simulink model "DRI_furnace"  (R2023b)
settings: Solver=ode15s  StartTime=0.0  StopTime=3600*24
values from neighbouring files (symbols this model uses):
  a_b = 6*(1-eps_bed)/(r_p*2)    (= 200)    [DRI_furnace_loader.m]
  A_furnace = pi*r_furnace^2    (= 23.7582944428)    [DRI_furnace_loader.m]
  A_furnace_pel = A_furnace*(1-eps_bed)    (= 11.8791472214)    [DRI_furnace_loader.m]
  A_wall = (2*pi*r_furnace*dz)    [DRI_furnace_loader.m]
  c_CH4init = interp1([1:1:length(c_CH4init)],c_CH4init, linspace(1,length(c_CH4init),n_furnace))    [DRI_furnace_loader.m]    (also in inital_conditions.m = out.CH4_conc.data(end,:); initcond.mat = [1.85705986545 1.89555733619 1.89749367615 1.89250716351 1.8; initcond_H2.mat = [-5.10200321778e-23 -5.14631233267e-23 -5.19105613109e-23 -5; initcond_NG.mat = [1.53547326032 1.50495486962 1.48970115024 1.4755028102 1.46)
  c_Cinit = interp1([1:1:length(c_Cinit)],c_Cinit, linspace(1,length(c_Cinit),n_furnace))    [DRI_furnace_loader.m]    (also in inital_conditions.m = out.C_conc.data(end,:); initcond.mat = [3.21457388191e-26 -1.33944556404e-26 -9.41053781484e-33 -9.; initcond_H2.mat = [-3.07981965757e-283 -7.05821276017e-284 -1.12151880238e-284; initcond_NG.mat = [40.5707549093 38.5039319297 36.8451113121 35.2570306703 33.)
  c_CO2init = interp1([1:1:length(c_CO2init)],c_CO2init, linspace(1,length(c_CO2init),n_furnace))    [DRI_furnace_loader.m]    (also in inital_conditions.m = out.CO2_conc.data(end,:); initcond.mat = [0.424855142623 0.487573768012 0.610878568601 0.778581871411; initcond_H2.mat = [8.08256932825e-22 8.11925418298e-22 8.15917924386e-22 8.201; initcond_NG.mat = [0.33936960913 0.362161667495 0.389241162314 0.417886502664 )
  c_COinit = interp1([1:1:length(c_COinit)],c_COinit, linspace(1,length(c_COinit),n_furnace))    [DRI_furnace_loader.m]    (also in inital_conditions.m = out.CO_conc.data(end,:); initcond.mat = [5.62429774676 5.68698007947 5.56998267729 5.3860363993 5.16; initcond_H2.mat = [-3.5707332813e-22 -3.59888147715e-22 -3.62743836785e-22 -3.; initcond_NG.mat = [7.01547259829 7.0384402498 7.00998897858 6.97797046171 6.94)
  c_Fe2O3init = interp1([1:1:length(c_Fe2O3init)],c_Fe2O3init, linspace(1,length(c_Fe2O3init),n_furnace))    [DRI_furnace_loader.m]    (also in inital_conditions.m = out.Fe2O3_conc.data(end,:); initcond.mat = [845.154140842 845.181508816 845.220501809 845.323312901 845; initcond_H2.mat = [-0.0380770099519 -0.0370367139242 -0.0360185883395 -0.03502; initcond_NG.mat = [-0.0405281021674 -0.0396025120519 -0.0386898228266 -0.03778)
  c_Fe3O4init = interp1([1:1:length(c_Fe3O4init)],c_Fe3O4init, linspace(1,length(c_Fe3O4init),n_furnace))    [DRI_furnace_loader.m]    (also in inital_conditions.m = out.Fe3O4_conc.data(end,:); initcond.mat = [826.123395955 826.094631755 826.211564736 834.377927258 899; initcond_H2.mat = [0.0321426182211 0.0314818734285 0.030826675132 0.0301767421; initcond_NG.mat = [0.0360465051239 0.0353534026747 0.0346647730928 0.033980211)
  c_Feinit = interp1([1:1:length(c_Feinit)],c_Feinit, linspace(1,length(c_Feinit),n_furnace))    [DRI_furnace_loader.m]    (also in inital_conditions.m = out.Fe_conc.data(end,:); initcond.mat = [836.997845525 830.524010614 758.675200979 644.11637995 545.; initcond_H2.mat = [2198.89990701 2151.53921086 2100.32127816 2045.76128409 198; initcond_NG.mat = [2217.04023267 2190.22219582 2162.02573698 2132.25158626 210)
  c_FeOinit = interp1([1:1:length(c_FeOinit)],c_FeOinit, linspace(1,length(c_FeOinit),n_furnace))    [DRI_furnace_loader.m]    (also in inital_conditions.m = out.FeO_conc.data(end,:); initcond.mat = [523.921847425 532.250412357 624.547839148 764.836368397 835; initcond_H2.mat = [239.269098944 300.197811145 366.088832018 436.279393422 510; initcond_NG.mat = [215.930334993 250.431267245 286.705532207 325.009485154 365)
  c_H2init = interp1([1:1:length(c_H2init)],c_H2init, linspace(1,length(c_H2init),n_furnace))    [DRI_furnace_loader.m]    (also in inital_conditions.m = out.H2_conc.data(end,:); initcond.mat = [8.579601171 8.64686368664 8.51185743267 8.39999947053 8.265; initcond_H2.mat = [17.2543528358 17.2782610911 17.296864644 17.3099892036 17.3; initcond_NG.mat = [11.1435961113 11.2383917061 11.232749456 11.2204098296 11.2)
  c_H2Oinit = interp1([1:1:length(c_H2Oinit)],c_H2Oinit, linspace(1,length(c_H2Oinit),n_furnace))    [DRI_furnace_loader.m]    (also in inital_conditions.m = out.H2O_conc.data(end,:); initcond.mat = [0.757633216435 0.883934685646 1.02867679163 1.11546273638 1; initcond_H2.mat = [0.442325343528 0.548013106661 0.662035872616 0.783558475201; initcond_NG.mat = [0.493575761349 0.511052154474 0.544598386657 0.580268512829)
  c_N2init = interp1([1:1:length(c_N2init)],c_N2init, linspace(1,length(c_N2init),n_furnace))    [DRI_furnace_loader.m]    (also in inital_conditions.m = out.N2_conc.data(end,:); initcond.mat = [0.304985476887 0.311307927602 0.311625933271 0.310806996864; initcond_H2.mat = [0.335892697728 0.338352501527 0.340869822099 0.343425499389; initcond_NG.mat = [0.34370092648 0.344898196415 0.344837358554 0.344718971495 )
  DRIflow = 45.1    [DRI_furnace_loader.m]
  dz = flip(diff(dzfun))    [DRI_furnace_loader.m]
  eps_bed = 0.5    [DRI_furnace_loader.m]
  MM_C = 12.011/1000    (= 0.012011)    [DRI_furnace_loader.m]
  MM_CH4 = 16.04    [DRI_furnace_loader.m]
  MM_CO = 28.01    [DRI_furnace_loader.m]
  MM_CO2 = 44.01    [DRI_furnace_loader.m]
  MM_Fe = 55.845/1000    (= 0.055845)    [DRI_furnace_loader.m]    (also in iron_props.m)
  MM_Fe2O3 = 159.69/1000    (= 0.15969)    [DRI_furnace_loader.m]    (also in iron_props.m)
  MM_Fe3O4 = 251.53/1000    (= 0.25153)    [DRI_furnace_loader.m]    (also in iron_props.m)
  MM_FeO = 71.844/1000    (= 0.071844)    [DRI_furnace_loader.m]    (also in iron_props.m)
  MM_Gan = 60.08/1000    (= 0.06008)    [DRI_furnace_loader.m]
  MM_H2 = 2.016    [DRI_furnace_loader.m]
  MM_H2O = 18.015    [DRI_furnace_loader.m]
  MM_N2 = 28.013    [DRI_furnace_loader.m]
  mol_Fe2O3init = rho_p*0.9665/MM_Fe2O3*V_s(2:end)    [DRI_furnace_loader.m]    (also in inital_conditions.m = out.mol_Fe2O3init.data(end,:); initcond.mat = [61783.2992712 61783.2992712 61783.2992712 61783.2992712 617)
  n_furnace = 25    [DRI_furnace_loader.m]
  ndotinit = interp1([1:1:length(ndotinit)],ndotinit, linspace(1,length(ndotinit),n_furnace))    [DRI_furnace_loader.m]    (also in inital_conditions.m = out.ndot.data(end,:); initcond.mat = [2210.71780913 2256.54672706 2258.85182304 2252.91568039 224; initcond_H2.mat = [2085.86199266 2093.15115329 2100.66626347 2108.33970255 211; initcond_NG.mat = [2330.74775425 2364.28126123 2378.87094646 2385.81987377 238)
  nr1init = ones(size(T_ginit))*33375    [DRI_furnace_loader.m]    (also in inital_conditions.m = out.nr1.data(end,:); initcond.mat = [61803.8716376 61802.685448 61800.9961847 61796.5422507 6178; initcond_H2.mat = [17138.8276975 17138.822469 17138.817352 17138.8123408 17138; initcond_NG.mat = [34277.6800528 34277.6707483 34277.6615734 34277.652487 3427)
  nr2init = ones(size(T_ginit))*22119    [DRI_furnace_loader.m]    (also in inital_conditions.m = out.nr2.data(end,:); initcond.mat = [41188.8753355 41188.8526513 41178.4232644 40740.5447947 379; initcond_H2.mat = [11425.7737029 11425.772508 11425.7713681 11425.7702806 1142; initcond_NG.mat = [22851.536777 22851.5353796 22851.5340375 22851.5327263 2285)
  nr3init = ones(size(T_ginit))*63083    [DRI_furnace_loader.m]    (also in inital_conditions.m = out.nr3.data(end,:); initcond.mat = [123566.152328 121180.275703 99887.5755955 72587.2577367 536; initcond_H2.mat = [31604.1937028 30923.4912249 30187.3497294 29403.1736897 285; initcond_NG.mat = [63729.8393954 62958.9426131 62148.4224578 61292.5508252 603)
  R = 8.314    [Bou.m]    (also in DRI_furnace_loader.m; G_CO.m; MD.m; SMR.m)
  r_furnace = 2.75    [DRI_furnace_loader.m]
  r_p = 15e-3/2    (= 0.0075)    [DRI_furnace_loader.m]
  Reducerflow = 2228.1*(x_H2in*MM_H2 + x_COin*MM_CO + x_H2Oin*MM_H2O +x_CO2in*MM_CO2 + x_N2in*MM_N2 + x_CH4in*MM_CH4)/1000    (= 31.1426394672)    [DRI_furnace_loader.m]
  rho_p = 3528    [DRI_furnace_loader.m]
  T_ginit = interp1([1:1:length(T_ginit)],T_ginit, linspace(1,length(T_ginit),n_furnace))    [DRI_furnace_loader.m]    (also in inital_conditions.m = out.T_g.data(end,:); initcond.mat = [1196.67659973 1106.80014704 1071.61124107 1050.32194229 103; initcond_H2.mat = [1206.04002008 1196.92003246 1187.72467669 1178.52571193 116; initcond_NG.mat = [1059.94701026 1050.97990802 1047.95611626 1045.20600654 104)
  T_sinit = interp1([1:1:length(T_sinit)],T_sinit, linspace(1,length(T_sinit),n_furnace))    [DRI_furnace_loader.m]    (also in inital_conditions.m = out.T_s.data(end,:); initcond.mat = [1154.91557113 1100.93660653 1069.19977285 1049.37027984 104; initcond_H2.mat = [1198.21532505 1188.90892541 1179.58573027 1170.31082456 116; initcond_NG.mat = [1055.14966191 1048.70059171 1045.82868823 1043.13322913 104)
  V_g = (4/3)*pi*r_p^3*n_pellets_dz*(eps_bed/(1-eps_bed))    [DRI_furnace_loader.m]
  V_p = 4/3*pi*r_p^3    (= 1.76714586764e-06)    [DRI_furnace_loader.m]
  V_s = (4/3)*pi*r_p^3*n_pellets_dz    [DRI_furnace_loader.m]
  x_CH4in = 0.105824828    [DRI_furnace_loader.m]
  x_CO2in = 0.024    [DRI_furnace_loader.m]
  x_COin = 0.320711862    [DRI_furnace_loader.m]
  x_H2in = 0.489526511    [DRI_furnace_loader.m]
  x_H2Oin = 0.042557156    [DRI_furnace_loader.m]
  x_N2in = 0.017379642    [DRI_furnace_loader.m]
libraries: simulink x1
(part 2 of 2)

== matlab function DRI_furnace/Subsystem/DRI Furnace ==
  data: Pin input; c_H2Oin input; c_H2in input; c_N2in input; c_COin input; c_CO2in input; c_CH4in input; u_gin input; T_gin input; ndotin input; rho_Fe2O3in input; rho_Fe3O4in input; rho_FeOin input; rho_Fein input; rho_Cin input; rho_Ganin input; u_s input; T_sin input; mol_Fe2O3in input; pellet_flow input; c_H2O input; c_H2 input; c_N2 input; c_CO input; c_CO2 input; c_CH4 input; rho_Fe2O3 input; rho_Fe3O4 input; rho_FeO input; rho_Fe input; rho_C input; T_s input; T_g input; nr1 input; nr2 input; nr3 input; ndot input; mol_Fe2O3 input; dcdt_H2O output; dcdt_H2 output; dcdt_N2 output; dcdt_CO output; dcdt_CO2 output; dcdt_CH4 output; drhodt_Fe2O3 output; drhodt_Fe3O4 output; drhodt_FeO output; drhodt_Fe output; drhodt_C output; dz parameter; n_furnace parameter; A_furnace parameter; r_p parameter; m_sin input; m_gin input; dTdt_s output; dTdt_g output; dnr1_dt output; dnr2_dt output; dnr3_dt output; dntot_dt output; dmolFe2O3_dt output; a_b parameter; rho_s output; mass_bal output; Cratio output; r_furnace parameter; A_wall parameter; A_furnace_pel parameter; eps_bed parameter; MM_H2O parameter; MM_H2 parameter; MM_N2 parameter; u_g output; P_g output; x_H2 output; x_H2O output; x_N2 output; MM_Fe2O3 parameter; MM_Fe3O4 parameter; MM_FeO parameter; MM_Fe parameter; R parameter; V_g parameter; V_s parameter; MM_CO parameter; MM_CO2 parameter; x_CO output; x_CO2 output; x_CH4 output; w_Fe2O3 output; w_Fe3O4 output; w_FeO output; w_Fe output; w_C output; w_Gan output; Xred output; v8 output; v9 output; m_s output; x1 output; x2 output; x3 output; m_g output; w_sum output; V_p parameter; MM_CH4 parameter; MM_Gan parameter; MM_C parameter
function [dcdt_H2O,dcdt_H2,dcdt_N2, dcdt_CO, dcdt_CO2, dcdt_CH4, drhodt_Fe2O3,drhodt_Fe3O4,drhodt_FeO,drhodt_Fe, drhodt_C, dTdt_s, dTdt_g, dnr1_dt,dnr2_dt,dnr3_dt, dntot_dt, dmolFe2O3_dt, rho_s, mass_bal, Cratio, u_g, P_g,x_H2, x_H2O, x_N2, x_CO, x_CO2, x_CH4, w_Fe2O3, w_Fe3O4, w_FeO, w_Fe, w_C, w_Gan, Xred, v8, v9, m_s, x1, x2, x3, m_g, w_sum]...
    = furnace(Pin, c_H2Oin,c_H2in,c_N2in,c_COin, c_CO2in, c_CH4in, u_gin,T_gin, ndotin, rho_Fe2O3in,rho_Fe3O4in,rho_FeOin,rho_Fein, rho_Cin, rho_Ganin, u_s, T_sin, mol_Fe2O3in, pellet_flow,...
                        c_H2O,c_H2,c_N2,c_CO, c_CO2, c_CH4, rho_Fe2O3,rho_Fe3O4,rho_FeO,rho_Fe,rho_C, T_s, T_g, nr1, nr2, nr3, ndot, mol_Fe2O3, dz,...
                        n_furnace, A_furnace, r_p, m_sin,m_gin, a_b, r_furnace, A_wall, A_furnace_pel, eps_bed, MM_H2O, MM_H2, MM_N2,MM_Fe2O3, MM_Fe3O4, MM_FeO, MM_Fe, R, V_g, V_s, MM_CO, MM_CO2, V_p, MM_CH4, MM_Gan, MM_C)

rho_Fe2O3(rho_Fe2O3<0) = 0;
rho_Fe3O4(rho_Fe3O4<0) = 0;
rho_FeO(rho_FeO<0) = 0;
rho_Fe(rho_Fe<0) = 0;
rho_C(rho_C<0) = 0;


c_H2(c_H2<0) = 0;
c_H2O(c_H2O<0) = 0;
c_N2(c_N2<0) = 0;
c_CO(c_CO<0) = 0;
c_CO2(c_CO2<0) = 0;
c_CH4(c_CH4<0) = 0;


H2O_diff_prop = [MM_H2O, 13.1];
H2_diff_prop = [MM_H2, 2.31*2];

CO_diff_prop = [MM_CO, 18.9];
CO2_diff_prop = [MM_CO2, 26.9];

nr1in = 0;
nr2in = 0;
nr3in = 0;


%Pin = 101325*2.40;

% initialize a lot of different variables the size of the spatial nodes
w_H2 = zeros(size(rho_Fe2O3));
w_H2O = zeros(size(rho_Fe2O3));
w_N2 = zeros(size(rho_Fe2O3));
w_CO = zeros(size(rho_Fe2O3));
w_CO2 = zeros(size(rho_Fe2O3));
w_CH4 = zeros(size(rho_Fe2O3));


x_H2 = zeros(size(rho_Fe2O3));
x_H2O = zeros(size(rho_Fe2O3));
x_N2 = zeros(size(rho_Fe2O3));
x_CO = zeros(size(rho_Fe2O3));
x_CO2 = zeros(size(rho_Fe2O3));
x_CH4 = zeros(size(rho_Fe2O3));


mu_g = zeros(size(rho_Fe2O3));
Cp_g = zeros(size(rho_Fe2O3));
Pr_g = zeros(size(rho_Fe2O3));

Cm_H2 = zeros(size(rho_Fe2O3));
Cm_H2O = zeros(size(rho_Fe2O3));

rho_g = zeros(size(rho_Fe2O3));

Nu = zeros(size(rho_Fe2O3));
Re_p = zeros(size(rho_Fe2O3));
Re_f = zeros(size(rho_Fe2O3));

k_g = zeros(size(rho_Fe2O3));
h_sg = zeros(size(rho_Fe2O3));
U_wall = zeros(size(rho_Fe2O3));

D_H2_H2O = zeros(size(rho_Fe2O3));
D_CO_CO2 = zeros(size(rho_Fe2O3));

k_diff_H2 = zeros(size(rho_Fe2O3));
k_diff_CO = zeros(size(rho_Fe2O3));


rho_s = zeros(size(rho_Fe2O3));

w_Fe2O3 = zeros(size(rho_Fe2O3));
w_Fe3O4 = zeros(size(rho_Fe2O3));
w_FeO = zeros(size(rho_Fe2O3));
w_Fe = zeros(size(rho_Fe2O3));
w_C = zeros(size(rho_Fe2O3));
w_Gan = zeros(size(rho_Fe2O3));
Cp_s = zeros(size(rho_Fe2O3));

x1 = zeros(size(rho_Fe2O3));
x2 = zeros(size(rho_Fe3O4));
x3 = zeros(size(rho_FeO));
Xred = zeros(size(rho_FeO));


x_COeq1 = zeros(size(rho_Fe2O3));
x_COeq2 = zeros(size(rho_Fe3O4));
x_COeq3 = zeros(size(rho_FeO));


%mol_Fe2O3 = zeros(size(rho_Fe2O3));
mol_Fe3O4 = zeros(size(rho_Fe3O4));
mol_FeO = zeros(size(rho_FeO));
mol_Fe = zeros(size(rho_FeO));
mol_C = zeros(size(rho_FeO));
Cratio = zeros(size(rho_FeO));

v1 = zeros(size(rho_Fe2O3));
v2 = zeros(size(rho_Fe3O4));
v3 = zeros(size(rho_FeO));

v4 = zeros(size(rho_Fe2O3));
v5 = zeros(size(rho_Fe3O4));
v6 = zeros(size(rho_FeO));
v7 = zeros(size(rho_FeO));
v8 = zeros(size(rho_FeO));
v9 = zeros(size(rho_FeO));
v10 = zeros(size(rho_FeO));

f1 = zeros(size(rho_Fe2O3));
f2 = zeros(size(rho_Fe3O4));
f3 = zeros(size(rho_FeO));

m_g = zeros(size(rho_Fe2O3));
m_s = zeros(size(rho_Fe2O3));

ct = zeros(size(rho_Fe2O3));

P_g = zeros(size(T_s));

%initializing each mass bal derivatives as zero to define size of each column vector
dcdt_H2O = zeros(size(c_H2O));
dcdt_H2 = zeros(size(c_H2));
dcdt_N2 = zeros(size(c_N2));
dcdt_CO = zeros(size(c_CO));
dcdt_CO2 = zeros(size(c_CO2));
dcdt_CH4 = zeros(size(c_CH4));

drhodt_Fe2O3 = zeros(size(rho_Fe2O3));
drhodt_Fe3O4 = zeros(size(rho_Fe3O4));
drhodt_FeO = zeros(size(rho_FeO));
drhodt_Fe = zeros(size(rho_Fe));
drhodt_C = zeros(size(rho_Fe));

dnr1_dt = zeros(size(rho_Fe2O3));
dnr2_dt = zeros(size(rho_Fe3O4));
dnr3_dt = zeros(size(rho_FeO));
dntot_dt = zeros(size(rho_FeO));
dmolFe2O3_dt = zeros(size(rho_FeO));

S_nr1 = zeros(size(rho_Fe2O3));
S_nr2 = zeros(size(rho_Fe3O4));
S_nr3 = zeros(size(rho_FeO));
S_ntot = zeros(size(rho_FeO));

u_g = zeros(size(rho_Fe2O3));

dTdt_s = zeros(size(T_s));
dTdt_g = zeros(size(T_g));

DelH1 = zeros(size(T_s));
DelH2 = zeros(size(T_s));
DelH3 = zeros(size(T_s));

DelH4 = zeros(size(T_s));
DelH5 = zeros(size(T_s));
DelH6 = zeros(size(T_s));

DelH7 = zeros(size(T_s));
DelH8 = zeros(size(T_s));




%% Inlet Gas and Iron Properties

% Weight fractions of each gas species

w_totin = (c_H2in*MM_H2 + c_H2Oin*MM_H2O + c_N2in*MM_N2 + c_COin*MM_CO + c_CO2in*MM_CO2 +  c_CH4in*MM_CH4);

w_H2in = c_H2in*MM_H2/w_totin;
w_H2Oin = c_H2Oin*MM_H2O /w_totin;
w_N2in = c_N2in*MM_N2/w_totin;
w_COin = c_COin*MM_CO/w_totin;
w_CO2in = c_CO2in*MM_CO2/w_totin;
w_CH4in = c_CH4in*MM_CH4/w_totin;


w_fracs = [w_H2in, w_H2Oin, w_N2in, w_COin, w_CO2in, w_CH4in]; % Create a vector of weight fractions for the prop_mix function

% Get properties from CoolProp interpolation based on temp of gas in
[rho_H2, mu_H2, k_H2, C_H2] = hydrogen(T_gin);
[rho_H2O, mu_H2O, k_H2O, C_H2O] = water(T_gin);
[rho_N2, mu_N2, k_N2, C_N2] = nitrogen(T_gin);
[rho_CO, mu_CO, k_CO, C_CO] = carbonmonoxide(T_gin);
[rho_CO2, mu_CO2, k_CO2, C_CO2] = carbondioxide(T_gin);
[rho_CH4, mu_CH4, k_CH4, C_CH4] = methane(T_gin);



% Create vectors of properties for prop_mix function
rhos = [rho_H2, rho_H2O, rho_N2, rho_CO, rho_CO2, rho_CH4];
mus = [mu_H2, mu_H2O, mu_N2, mu_CO, mu_CO2, mu_CH4];
ks = [k_H2, k_H2O, k_N2, k_CO, k_CO2, k_CH4];
Cps = [C_H2, C_H2O, C_N2, C_CO, C_CO2, C_CH4];

% get vicosicty and specific heat of gas mixture in
[~, mu_gin, ~,  Cp_gin] = prop_mix(rhos, mus, ks, Cps, w_fracs);

% density of gas coming from ideal gas law
rho_gin = ((c_H2in*MM_H2 + c_H2Oin*MM_H2O + c_N2in*MM_N2 + c_COin*MM_CO + c_CO2in*MM_CO2 + c_CH4in*MM_CH4 )/1000); %kg/m^3 of gas

% density of the iron pellets
rho_sin = rho_Fe2O3in + rho_Fe3O4in + rho_FeOin + rho_Fein + rho_Cin + rho_Ganin; %kg/m^3 of pellet in to the reactor

% weight fraction of each iron species at each spatial node
w_Fe2O3in =  rho_Fe2O3in/rho_sin;
w_Fe3O4in =  rho_Fe3O4in/rho_sin;
w_FeOin =  rho_FeOin/rho_sin;
w_Fein =  rho_Fein/rho_sin;
w_Cin =  rho_Cin/rho_sin;
w_Ganin =  rho_Ganin/rho_sin;



% specific heat of each iron species as a funciton of temperature of the solids
[Cps_iron, ~] = iron_props(T_sin); %J/kg-K, specific heat

% vector of weight fractions for mass weithed average
w_iron = [w_Fe2O3in, w_Fe3O4in, w_FeOin, w_Fein, w_Cin, w_Ganin];
Cp_sin = dot(Cps_iron, w_iron); %J/kg-K, mass weighted average of specific heat


%% Spatial Gas and Iron Properties 

for i = 1:n_furnace
    
    w_tot = (c_H2(i)*MM_H2 + c_H2O(i)*MM_H2O + c_N2(i)*MM_N2 + c_CO(i)*MM_CO + c_CO2(i)*MM_CO2 + c_CH4(i)*MM_CH4);

    % Weight fractions of each gas species for each spatial node
    w_H2(i) = c_H2(i)*MM_H2/w_tot;
    w_H2O(i) = c_H2O(i)*MM_H2O /w_tot; 
    w_N2(i) = c_N2(i)*MM_N2/w_tot; 
    w_CO(i) = c_CO(i)*MM_CO/w_tot;
    w_CO2(i) = c_CO2(i)*MM_CO2/w_tot;
    w_CH4(i) = c_CH4(i)*MM_CH4/w_tot;


    % density using molar concentrations
    rho_g(i) = ((c_H2(i)*MM_H2 + c_H2O(i)*MM_H2O + c_N2(i)*MM_N2 + c_CO(i)*MM_CO + c_CO2(i)*MM_CO2 + c_CH4(i)*MM_CH4)/1000); % kg/m^3 of gas, density of gas
    
    % mole fractions of each gas species for each spatial node
    ct(i) = c_H2(i) + c_H2O(i) + c_N2(i) + c_CO(i) + c_CO2(i) + c_CH4(i);
    x_H2(i) = c_H2(i)/ct(i);
    x_H2O(i) = c_H2O(i)/ct(i);
    x_N2(i) = c_N2(i)/ct(i);
    x_CO(i) = c_CO(i)/ct(i);
    x_CO2(i) = c_CO2(i)/ct(i);
    x_CH4(i) = c_CH4(i)/ct(i);
    
    % Create vectors of weight frac for prop_mix function
    w_fracs = [w_H2(i), w_H2O(i), w_N2(i), w_CO(i), w_CO2(i), w_CH4(i)];

    % Get properties from CoolProp interpolation based on temp of gas at each spatial node
    [rho_H2, mu_H2, k_H2, C_H2] = hydrogen(T_g(i));
    [rho_H2O, mu_H2O, k_H2O, C_H2O] = water(T_g(i));
    [rho_N2, mu_N2, k_N2, C_N2] = nitrogen(T_g(i));
    [rho_CO, mu_CO, k_CO, C_CO] = carbonmonoxide(T_gin);
    [rho_CO2, mu_CO2, k_CO2, C_CO2] = carbondioxide(T_gin);
    [rho_CH4, mu_CH4, k_CH4, C_CH4] = methane(T_gin);

    Cm_H2(i) = C_H2*MM_H2/1000;
    Cm_H2O(i) = C_H2O*MM_H2O/1000;
    
    % Create vectors of properties for prop_mix function
    rhos = [rho_H2, rho_H2O, rho_N2, rho_CO, rho_CO2, rho_CH4];
    mus = [mu_H2, mu_H2O, mu_N2, mu_CO, mu_CO2, mu_CH4];
    ks = [k_H2, k_H2O, k_N2, k_CO, k_CO2, k_CH4];
    Cps = [C_H2, C_H2O, C_N2, C_CO, C_CO2, C_CH4];

    % get vicosicty, thermal conductivity, specific heat of gas mixture at each spatial node
    [~, mu_g(i), k_g(i), Cp_g(i)] = prop_mix(rhos, mus, ks, Cps, w_fracs);
    
    % density of the iron pellets
    rho_s(i) = rho_Fe2O3(i) + rho_Fe3O4(i) + rho_FeO(i) + rho_Fe(i) + rho_C(i) + rho_Ganin; %kg/m^3 of pellet
    
    % weight fraction of each iron species at each spatial node
    w_Fe2O3(i) =  rho_Fe2O3(i)/rho_s(i);
    w_Fe3O4(i) =  rho_Fe3O4(i)/rho_s(i);
    w_FeO(i) =  rho_FeO(i)/rho_s(i);
    w_Fe(i) =  rho_Fe(i)/rho_s(i);
    w_C(i) =  rho_C(i)/rho_s(i);
    w_Gan(i) =  rho_Ganin/rho_s(i);

    % specific heat of each iron species as a funciton of temperature of the solids
    [Cps_iron, ~] = iron_props(T_s(i)); %J/kg-K, specific heat
    
    % vector of weight fractions for mass weithed average
    w_iron = [w_Fe2O3(i), w_Fe3O4(i), w_FeO(i), w_Fe(i), w_C(i), w_Gan(i)];
    Cp_s(i) = dot(Cps_iron, w_iron); %J/kg-K, mass weighted average of specific heat

end

x_sum = x_H2 + x_H2O + x_N2 + x_CO + x_CO2 + x_CH4;
w_sum = w_Fe2O3 + w_Fe3O4 + w_FeO + w_Fe + w_C + w_Gan;

%ndot = zeros(size(T_g_plot));

%% Spatial Gas Velocity and Pressure

for i = 1:n_furnace
    
    if  i == 1

        u_gin = (ndotin*R*T_gin)/(Pin*eps_bed*A_furnace); % m/s, interstitial gas flow in

        % average properties for Ergun eq.
        mu_gavg = (mu_gin + mu_g(i))/2;
        rho_gavg = (rho_gin + rho_g(i))/2;
        
        %P drop using Ergun equation and velocicty at node upwind
        P_g(i) = -((150*(1-eps_bed)^2*mu_gavg*u_gin)/((2*r_p)^2*eps_bed^2)+(1.75*rho_gavg*(1-eps_bed)*u_gin^2)/(2*r_p*eps_bed))*dz(i) + Pin; % Pa, pressure of gas at node 1
        
        % velocity using ideal gas law coupled with Ergun eq. 
        u_g(i) = (ndot(i)*R*T_g(i))/(P_g(i)*eps_bed*A_furnace); % m/s, interstitial gas flow in
        
    else
      
        % average properties for Ergun eq.
        mu_gavg = (mu_g(i-1) + mu_g(i))/2;
        rho_gavg = (rho_g(i-1) + rho_g(i))/2;

        %P drop using Ergun equation and velocicty at node upwind
        P_g(i) = -((150*(1-eps_bed)^2*mu_gavg*u_g(i-1))/((2*r_p)^2*eps_bed^2)+(1.75*rho_gavg*(1-eps_bed)*u_g(i-1)^2)/(2*r_p*eps_bed))*dz(i) + P_g(i-1);
        P_g(P_g<0.25*101325) = 0.25*101325; %just helps fix errors at begining of sims.
 
        % velocity using ideal gas law coupled with Ergun eq. 
        u_g(i) = (ndot(i)*R*T_g(i))/(P_g(i)*eps_bed*A_furnace); % m/s, interstitial gas flow in

    end

end

%% Heat and Mass Transfer Coefficients

for i = 1:n_furnace
    Pr_g(i) = Cp_g(i)*mu_g(i)/k_g(i); % unitless, Prandlt number of gas

    Re_p(i) = (rho_g(i)*u_g(i)*2*r_p)/mu_g(i); % unitless, Reynolds number of gas using pellet diameter as characteristic length
    Re_f(i) = (rho_g(i)*u_g(i)*2*r_furnace)/mu_g(i); % unitless, Reynolds number of gas furnace diameter as characteristic length
    
    Nu(i) = 2 + 0.39*Re_p(i)^(1/2)*Pr_g(i)^(1/3); % unitless, Nusselt number of heat transfer from gas to solid
    h_sg(i) = Nu(i)*k_g(i)/(2*r_p); % W/m^2-K, convective heat transfer coeffient of solid to gas
 
    U_wall(i) = (2.26 * Re_p(i)^0.8*Pr_g(i)^(1/3)*exp((-12*r_p)/(2*r_furnace)))*((mu_g(i)/rho_g(i))/(2*r_furnace));% W/m^2-K, convective heat transfer coeffient of gas to wall
    %U_wall(i) = (2.26 * Re_p(i)^0.8*Pr_g(i)^(1/3)*exp((-12*r_p)/(2*r_furnace)))*((k_g(i))/(2*r_furnace));
    %U_wall(i) = (0.023*Re_f(i)^0.8*Pr_g(i)^(0.3))*((k_g(i))/(2*r_furnace));

    D_H2_H2O(i) = fuller(H2O_diff_prop, H2_diff_prop, T_g(i), P_g(i)); % m^2/s, diffusion coefficent of H2O/H2 at gas temp and pressure for each spatial node
    D_CO_CO2(i) = fuller(CO_diff_prop, CO2_diff_prop, T_g(i), P_g(i)); % m^2/s, diffusion coefficent of H2O/H2 at gas temp and pressure for each spatial node
    
    mu_kine = mu_g(i)/rho_g(i); %m^2/2, kinematic viscosity of gas
    
    Sc = mu_kine/D_H2_H2O(i); % unitless, Schmidt number
    Sh = 2 + 0.39*Re_p(i)^(1/2)*Sc^(1/3); % unitless, Sherwood number of diffusion of gas to pellet film
    
    k_diff_H2(i) = Sh*D_H2_H2O(i)/(2*r_p); % m/s, mass tranfer coefficient of gas to pellet
    k_diff_CO(i) = Sh*D_CO_CO2(i)/(2*r_p); % m/s, mass tranfer coefficient of gas to pellet

end
Pr_g;
Re_p;

%% Reaction Progress in a pellets

x_CO_ogs = zeros(size(c_N2));

%% Rate of Reaction using Unreacted Shrinking Core Model

for i = 1:n_furnace
  
    % find moles of each iron species available for reaction
    %mol_Fe2O3 = rho_Fe2O3in/MM_Fe2O3*A_furnace_pel.*dz(2:end)'; %moles
    
    %mol_Fe2O3(i) = rho_Fe2O3in/MM_Fe2O3*V_s(i+1);
    mol_Fe3O4(i) = mol_Fe2O3(i)*(2/3); % 2/3 from stoichiometry 
    mol_FeO(i) = mol_Fe3O4(i)*(3/1); % 3/1 from stoichiometry
    mol_Fe(i) = mol_FeO(i); %1/1 from stoichiometry
    mol_C(i) = rho_C(i)/MM_C*V_s(i+1);

    % f values are fraction of moles that have reacted for each nr which is moles reacted down the length of the reactor
    f1(i) = nr1(i)/mol_Fe2O3(i);
    f2(i) = nr2(i)/mol_Fe3O4(i);
    f3(i) = nr3(i)/mol_FeO(i);
    
    % fraction of moles available to react
    a = 1-f1(i);
    b = 1-f2(i);
    c = 1-f3(i);
    
    % make sure we aren't slighlty negative from rounding etc. as this will cause errors
    a(a<1e-15) = 1e-15;
    b(b<1e-15) = 1e-15;
    c(c<1e-15) = 1e-15;
    
    % x values are used in the unreacted shrinking core model (USCM)
    % x values are the radius of unreacted iron species for each reaction
    % x values of zero mean that that iron reaction has fully reacted
    % the 1/3 comes from geometry of a sphere
    x1(i) = (a).^(1/3); % radius of Fe3O4/Fe2O3
    x2(i) = (b).^(1/3); % radius of FeO/Fe3O4
    x3(i) = (c).^(1/3); % radisu of Fe/FeO

    Xred(i) = 1 -((1/9)*x1(i) + (2/9)*x1(i) + (6/9)*x3(i)); 
    %Xred(i) =  w_Fe(i)/w_sum(i);

    x_H2_ogs = 1 - x_CO(i) - x_CO2(i) - x_N2(i);
    x_CO_ogs(i) = 1 - x_H2(i) - x_H2O(i) - x_N2(i);
    % 
    % tol = 1e-5;
    % if x1(i) < tol && x2(i) < tol
    %     rxns = 1;
    % elseif x2(i) < tol
    %     rxns = 2;
    % else
    %     rxns = 3;
    % end
    rxns = 3;
   

    %Rate of reaction for three seperate reactions 1, 2, 3 using unreacted
    %shrinking core model in mol H2 per s per pellet
    [v1(i), v2(i), v3(i)] = USCM(x1(i),x2(i),x3(i), r_p, T_s(i), c_H2(i), ct(i), x_H2_ogs, rxns, k_diff_H2(i)); %mol H2 per s per pellet
    [v4(i), v5(i), v6(i), x_COeq1(i), x_COeq2(i), x_COeq3(i)] = USCM_CO(x1(i),x2(i),x3(i), r_p, T_s(i), c_CO(i), ct(i), x_CO_ogs(i), rxns, k_diff_CO(i)); %mol H2 per s per pellet
    
    v7(i) = WGS(Xred(i), T_g(i), P_g(i), V_p, x_H2(i), x_H2O(i), x_CO(i), x_CO2(i));
    %v7(i) = 0;
    v8(i) = SMR(Xred(i), T_g(i), P_g(i), V_p, x_H2(i), x_H2O(i), x_CO(i), x_CH4(i));
    
    Cratio(i) = (w_C(i)/(MM_C))/(w_Fe(i)/MM_Fe); 
    v9(i) = MD(T_s(i), P_g(i), x_H2(i), x_CH4(i), Cratio(i), eps_bed);
    %v10(i) = Bou(T_s(i), P_g(i), x_H2(i), x_CO(i), x_CO2(i), Cratio(i), eps_bed);

    %v10(i) = 0;
    %v9(i) = 0;
    % v1(i) = 0;
    % v2(i) = 0;
    % v3(i) = 0;
    % v4(i) = 0;
    % v5(i) = 0;
    % v6(i) = 0;
    v7(i) = 0;
    v8(i) = 0;
    v9(i) = 0;


end

% sometimes will get small negative values which cause problems so set those to zero
v1(v1<0) = 0;
v2(v2<0) = 0;
v3(v3<0) = 0;
v4(v4<0) = 0;
v5(v5<0) = 0;
v6(v6<0) = 0;

%v10(v10<0) = 0;
%v9(v9<0) = 0;



%v8(v8>0) = 0;

tol = 10;
v1(v1>tol) = tol;
v2(v2>tol) = tol;
v3(v3>tol) = tol;
v4(v4>tol) = tol;
v5(v5>tol) = tol;
v6(v6>tol) = tol;

%v7(i) = 0;


v7(v7>tol) = tol;
v7(v7<-tol) = -tol;
% 
% tol = 1e-3;
% v8(v8>tol) = tol;
% v8(v8<-tol) = -tol;

%% Source Terms from Reaction
A_furnace_gas = A_furnace*eps_bed;

% Source terms of each gas from reactions -- mol/m^3 gas*s
S_H2O = (v1 + v2 + v3 - v7 + v8)*(pellet_flow/(A_furnace_pel*u_s))*((1-eps_bed)/eps_bed); %mol/m^3 gas *s
S_H2 = (-v1 - v2 - v3 + v7 - 3*v8 + 2*v9)*(pellet_flow/(A_furnace_pel*u_s))*((1-eps_bed)/eps_bed); %mol/m^3 gas *s


% Source terms of each gas from reactions -- mol/m^3 gas*s
S_CO2 = (v4 + v5 + v6 + v7 + v10)*(pellet_flow/(A_furnace_pel*u_s))*((1-eps_bed)/eps_bed); %mol/m^3 gas *s
S_CO = (-v4 - v5 - v6 - v7 - v8 -2*v10)*(pellet_flow/(A_furnace_pel*u_s))*((1-eps_bed)/eps_bed); %mol/m^3 gas *s

S_CH4 = (v8 - v9)*(pellet_flow/(A_furnace_pel*u_s))*((1-eps_bed)/eps_bed); %mol/m^3 gas *s


% Source terms of each iron species : note that molar masses are in kg/mol 
S_Fe2O3 = -3*MM_Fe2O3*(v1+v4) * (pellet_flow/(A_furnace_pel*u_s)); % kg/m^3 solid*s
S_Fe3O4 = MM_Fe3O4*(2*(v1+v4) - (v2+v5)) * (pellet_flow/(A_furnace_pel*u_s));  % kg/m^3 solid*s
S_FeO = MM_FeO*(3*(v2+v5) - (v3+v6))* (pellet_flow/(A_furnace_pel*u_s));  % kg/m^3 solid*s
S_Fe = MM_Fe*(v3+v6) * (pellet_flow/(A_furnace_pel*u_s)); % kg/m^3 solid*s
S_C = MM_C*(v9+v10)*(pellet_flow/(A_furnace_pel*u_s)); %kg/m^3 solid *s


S_ntot = (-2*v8 + 2*v9- v10)*(pellet_flow)*((1-eps_bed)/eps_bed); %mol/s^2

for i = 1:n_furnace
    % Source terms of each moles of iron species reacted!
    S_nr1(i) = 3*(v1(i)+v4(i))*(pellet_flow*dz(i+1)/u_s); % moles Fe2O3 reacted
    S_nr2(i) = (v2(i)+v5(i))*(pellet_flow*dz(i+1)/u_s);  % moles Fe3O4 reacted
    S_nr3(i) = (v3(i)+v6(i))*(pellet_flow*dz(i+1)/u_s); % moles FeO reacted
end

%% Mass Balances
%Accounts for advective transport and reaction

%Mass balance equations - 

for i = 1:n_furnace
    
    if  i == 1
        
        % change in concentrtation of each gas species, mol/m^3-s
        dcdt_H2O(i) = (u_gin*c_H2Oin - u_g(i)*c_H2O(i))/dz(i) + S_H2O(i);
        dcdt_H2(i) = (u_gin*c_H2in - u_g(i)*c_H2(i))/dz(i) + S_H2(i);
        dcdt_N2(i) = (u_gin*c_N2in - u_g(i)*c_N2(i))/dz(i);
        dcdt_CO(i) = (u_gin*c_COin - u_g(i)*c_CO(i))/dz(i) + S_CO(i);
        dcdt_CO2(i) = (u_gin*c_CO2in - u_g(i)*c_CO2(i))/dz(i) + S_CO2(i);
        dcdt_CH4(i) = (u_gin*c_CH4in - u_g(i)*c_CH4(i))/dz(i) + S_CH4(i);


        m_g(i) = rho_g(i)*V_g(i)*u_g(i)/dz(i); % kg/s, mass flow rate of gas

        dntot_dt(i) = (u_gin*ndotin - u_g(i)*ndot(i))/dz(i) + S_ntot(i);


    else
     
        % change in concentrtation of each gas species, mol/m^3-s
        dcdt_H2O(i) = (u_g(i-1)*c_H2O(i-1) - u_g(i)*c_H2O(i))/dz(i) + S_H2O(i);
        dcdt_H2(i) = (u_g(i-1)*c_H2(i-1) - u_g(i)*c_H2(i))/dz(i) + S_H2(i);
        dcdt_N2(i) = (u_g(i-1)*c_N2(i-1) - u_g(i)*c_N2(i))/dz(i);
        dcdt_CO(i) = (u_g(i-1)*c_CO(i-1) - u_g(i)*c_CO(i))/dz(i) + S_CO(i);
        dcdt_CO2(i) = (u_g(i-1)*c_CO2(i-1) - u_g(i)*c_CO2(i))/dz(i) + S_CO2(i);
        dcdt_CH4(i) = (u_g(i-1)*c_CH4(i-1) - u_g(i)*c_CH4(i))/dz(i) + S_CH4(i);

        m_g(i) = rho_g(i)*V_g(i)*u_g(i)/dz(i); % kg/s, mass flow rate of gas

        dntot_dt(i) = (u_g(i-1)*ndot(i-1) - u_g(i)*ndot(i))/dz(i) + S_ntot(i);


    end

end


for i = 1:n_furnace

    if i == n_furnace

        % change in solid mass concentration in kg/m^3-s
        %Fe2O3
        drhodt_Fe2O3(i) = (u_s/dz(i+1))*(rho_Fe2O3in - rho_Fe2O3(i)) + S_Fe2O3(i);
        %Fe3O4
        drhodt_Fe3O4(i) = (u_s/dz(i+1))*(rho_Fe3O4in - rho_Fe3O4(i)) + S_Fe3O4(i);
        %FeO
        drhodt_FeO(i) = (u_s/dz(i+1))*(rho_FeOin - rho_FeO(i)) + S_FeO(i);
        %Fe
        drhodt_Fe(i) = (u_s/dz(i+1))*(rho_Fein - rho_Fe(i)) + S_Fe(i); 
        %C
        drhodt_C(i) = (u_s/dz(i+1))*(rho_Cin - rho_C(i)) + S_C(i); 

        dmolFe2O3_dt(i) = (u_s/dz(i+1))*(mol_Fe2O3in - mol_Fe2O3(i));

       
        m_s(i) = rho_s(i)*V_s(i+1)*u_s/dz(i+1); % kg/s, mass flow rate of solid

    else

        % change in solid mass concentration in kg/m^3-s
        %Fe2O3
        drhodt_Fe2O3(i) = (u_s/dz(i+1))*(rho_Fe2O3(i+1) - rho_Fe2O3(i)) + S_Fe2O3(i);
        %Fe3O4
        drhodt_Fe3O4(i) = (u_s/dz(i+1))*(rho_Fe3O4(i+1) - rho_Fe3O4(i)) + S_Fe3O4(i);
        %FeO
        drhodt_FeO(i) = (u_s/dz(i+1))*(rho_FeO(i+1) - rho_FeO(i)) + S_FeO(i);
        %Fe
        drhodt_Fe(i) = (u_s/dz(i+1))*(rho_Fe(i+1) - rho_Fe(i)) + S_Fe(i);
        %C
        drhodt_C(i) = (u_s/dz(i+1))*(rho_C(i+1) - rho_C(i)) + S_C(i); 

        dmolFe2O3_dt(i) = (u_s/dz(i+1))*(mol_Fe2O3(i+1) - mol_Fe2O3(i));
        
        m_s(i) = rho_s(i)*V_s(i+1)*u_s/dz(i+1); % kg/s, mass flow rate of solid

    end

end


for i = 1:n_furnace

    if i == n_furnace
        % mole/s reacted from each iron reaction
        %nr1
        dnr1_dt(i) = (u_s/dz(i+1))*(nr1in - nr1(i)) + S_nr1(i);
        %nr2
        dnr2_dt(i) = (u_s/dz(i+1))*(nr2in - nr2(i)) + S_nr2(i);
        %nr3
        dnr3_dt(i) = (u_s/dz(i+1))*(nr3in - nr3(i)) + S_nr3(i);


    else
        
        % mole/s reacted from each iron reaction
        %nr1
        dnr1_dt(i) = (u_s/dz(i+1))*(nr1(i+1) - nr1(i)) + S_nr1(i);
        %nr2
        dnr2_dt(i) = (u_s/dz(i+1))*(nr2(i+1) - nr2(i)) + S_nr2(i);
        %nr3
        dnr3_dt(i) = (u_s/dz(i+1))*(nr3(i+1) - nr3(i)) + S_nr3(i);

    end
end


% Mass balance checks all in kg/s
m_gout = (c_H2(end)*(MM_H2/1000) + c_H2O(end)*(MM_H2O/1000)+c_N2(end)*(MM_N2/1000) + c_CO(end)*(MM_CO/1000) + c_CO2(end)*(MM_CO2/1000))*u_g(end)*A_furnace_gas;
m_sout = (rho_Fe2O3(1) + rho_Fe3O4(1) + rho_FeO(1) + rho_Fe(1) + rho_C(1) + rho_Ganin)*u_s*A_furnace_pel;
m_gout = m_g(end);
mass_in = m_gin + m_sin;
mass_out = m_gout + m_sout;

mass_bal = mass_in - mass_out;


%% Energy Balance

T_amb = 25+273;

for i = 1:n_furnace
    
    % heats of reaction for each reaction, J/mol H2
    % comes from regression lines based on heat of reaction from heat_rxn function
    % DelH1(i) = 8e-9*T_s(i)^4 - 4e-5*T_s(i)^3 + 0.0428*T_s(i)^2 - 13.082*T_s(i) - 5779.4;
    % DelH2(i) = -0.0326*T_s(i)^2 + 5.6049*T_s(i) + 63394;
    % DelH3(i) = 0.0141*T_s(i)^2 - 31.892*T_s(i) + 38460;
    % 
    % DelH4(i) = 1e-8*T_s(i)^4 - 6e-5*T_s(i)^3 + 0.08222*T_s(i)^2 - 27.272*T_s(i) - 45311;
    % DelH5(i) = -0.032*T_s(i)^2 + 14.505*T_s(i) + 19120;
    % DelH6(i) = 0.0146*T_s(i)^2 - 22.992*T_s(i) - 5813.9;

    DelH1(i) = 18437.9 -102.28*T_s(i) + 0.097044*T_s(i)^2;
    DelH2(i) = 52360.5 +73.29*T_s(i) - 0.097044*T_s(i)^2;
    DelH3(i) = 40087.4 -44.66*T_s(i) + 0.023847*T_s(i)^2;

    DelH4(i) = -26177.6 -92.125*T_s(i) + 0.096808*T_s(i)^2;
    DelH5(i)  = 7744.5 +83.5404*T_s(i) - 0.09669*T_s(i)^2;
    DelH6(i) = -4527.4 -34.5157*T_s(i) + 0.023612*T_s(i)^2;
    
    DelH7(i) = (-10000 + 2.31*(T_g(i) -273))*4.184;
    DelH8(i) = (-45200 - 16.59*T_g(i) + 9.46e-3*T_g(i)^2)*4.184;

    if i == 1
        % K/s, temp change of solid and gas
        dTdt_s(i) = (m_s(i+1)*Cp_s(i+1))/(rho_s(i)*Cp_s(i)*V_s(i+1))*T_s(i+1) - m_s(i)/(rho_s(i)*V_s(i+1))*T_s(i)...   
        - ((h_sg(i)*3)/(rho_s(i)*Cp_s(i)*r_p))*(T_s(i)-T_g(i)) + ...
          (1/(rho_s(i)*Cp_s(i)))*(-v1(i)*DelH1(i) -v2(i)*DelH2(i) -v3(i)*DelH3(i) - v4(i)*DelH4(i) -v5(i)*DelH5(i) -v6(i)*DelH6(i) - v7(i)*DelH7(i) - v8(i)*DelH8(i))*(pellet_flow/(A_furnace_pel*u_s));
       
       dTdt_g(i) = (m_gin*Cp_gin)/(rho_g(i)*Cp_g(i)*V_g(i))*T_gin - m_g(i)/(rho_g(i)*V_g(i))*T_g(i)...   
        - ((h_sg(i)*a_b)/(rho_g(i)*Cp_g(i)*eps_bed))*(T_g(i)-T_s(i))...
        - ((U_wall(i)*A_wall(i))/(rho_g(i)*Cp_g(i)*V_g(i)))*(T_g(i)-T_amb) ;


    elseif i == n_furnace
        
        % K/s, temp change of solid and gas
        dTdt_s(i) = (m_sin*Cp_sin)/(rho_s(i)*Cp_s(i)*V_s(i+1))*T_sin - m_s(i)/(rho_s(i)*V_s(i+1))*T_s(i)...   
        - ((h_sg(i)*3)/(rho_s(i)*Cp_s(i)*r_p))*(T_s(i)-T_g(i)) + ... 
          (1/(rho_s(i)*Cp_s(i)))*(-v1(i)*DelH1(i) -v2(i)*DelH2(i) -v3(i)*DelH3(i) - v4(i)*DelH4(i) -v5(i)*DelH5(i) -v6(i)*DelH6(i)  - v7(i)*DelH7(i) - v8(i)*DelH8(i))*(pellet_flow/(A_furnace_pel*u_s));
       
        dTdt_g(i) = (m_g(i-1)*Cp_g(i-1))/(rho_g(i)*Cp_g(i)*V_g(i))*T_g(i-1) - m_g(i)/(rho_g(i)*V_g(i))*T_g(i)...   
          - ((h_sg(i)*a_b)/(rho_g(i)*Cp_g(i)*eps_bed))*(T_g(i)-T_s(i))...
          - ((U_wall(i)*A_wall(i))/(rho_g(i)*Cp_g(i)*V_g(i)))*(T_g(i)-T_amb);


    else
        
        % K/s, temp change of solid and gas
        dTdt_s(i) = (m_s(i+1)*Cp_s(i+1))/(rho_s(i)*Cp_s(i)*V_s(i+1))*T_s(i+1) - m_s(i)/(rho_s(i)*V_s(i+1))*T_s(i)...   
        - ((h_sg(i)*3)/(rho_s(i)*Cp_s(i)*r_p))*(T_s(i)-T_g(i))+ ...
          (1/(rho_s(i)*Cp_s(i)))*(-v1(i)*DelH1(i) -v2(i)*DelH2(i) -v3(i)*DelH3(i) - v4(i)*DelH4(i) -v5(i)*DelH5(i) -v6(i)*DelH6(i) - v7(i)*DelH7(i) - v8(i)*DelH8(i))*(pellet_flow/(A_furnace_pel*u_s));
        
        dTdt_g(i) = (m_g(i-1)*Cp_g(i-1))/(rho_g(i)*Cp_g(i)*V_g(i))*T_g(i-1) - m_g(i)/(rho_g(i)*V_g(i))*T_g(i)...   
        - ((h_sg(i)*a_b)/(rho_g(i)*Cp_g(i)*eps_bed))*(T_g(i)-T_s(i))...
        - ((U_wall(i)*A_wall(i))/(rho_g(i)*Cp_g(i)*V_g(i)))*(T_g(i)-T_amb);


    end

end

dTdt_s = zeros(size(rho_Fe));
dTdt_g = zeros(size(rho_Fe));


Q_g = (m_gin*Cp_gin*T_gin)/1e6;
P_g = P_g./101325;

% Energy balance check, MW
% changing Cps - counter-current
q_g = (m_gout*Cp_g(end)*T_g(end) - m_gin*Cp_gin*T_gin)/1e6;
q_s = (m_sout*Cp_s(1)*T_s(1) - m_sin*Cp_sin*T_sin)/1e6;


end

== matlab function DRI_furnace/solid_conc ==
  data: rho_Fe2O3in output; w_Fe2O3 input; w_Fe3O4 input; w_FeO input; w_Fe input; w_C input; w_Gan input; m_solid input; rho_Fe3O4in output; rho_FeOin output; A_furnace parameter; rho_Fein output; rho_Cin output; rho_Ganin output; u_sin output; rho_p parameter; eps_bed parameter; pellet_flow output; r_p parameter; rho_bedin output; mol_Fe2O3in output; V_s parameter; MM_Fe2O3 parameter
function [rho_Fe2O3in, rho_Fe3O4in, rho_FeOin, rho_Fein, rho_Cin, rho_Ganin, u_sin, pellet_flow, rho_bedin, mol_Fe2O3in] = solid_conc(w_Fe2O3, w_Fe3O4, w_FeO, w_Fe, w_C, w_Gan, m_solid, A_furnace,rho_p, eps_bed, r_p, V_s, MM_Fe2O3)

%toal mass concentration using ped porosity and density of pellet
rho_bedin = rho_p; %kg/^3 of SOLID

%mass concentrations of each iron species in
rho_Fe2O3in = rho_bedin * w_Fe2O3; %kg/m^3 of pellet
rho_Fe3O4in = rho_bedin * w_Fe3O4; %kg/m^3 of pellet
rho_FeOin = rho_bedin * w_FeO; %kg/m^3 of pellet
rho_Fein = rho_bedin * w_Fe; %kg/m^3 of pellet
rho_Cin = rho_bedin * w_C; %kg/m^3 of pellet
rho_Ganin = rho_bedin * w_Gan; %kg/m^3 of pellet

mol_Fe2O3in = rho_Fe2O3in/MM_Fe2O3*V_s(end);

%vol_flow = m_solid/(rho_bedin*(1-eps_bed)); %m^3 total/s

u_sup = m_solid/(rho_p*A_furnace);%*(1-eps_bed));

            
u_sin = u_sup/(1-eps_bed);

%interstitial velocity of mass flow, m/s
%u_sin = m_solid/rho_bedin/(A_furnace*(1-eps_bed));


%check this!
pellet_flow = (3*m_solid)/(4*pi*r_p^3*rho_bedin); %pellets/s
